simulink model "array_sum"  (R2013b)
settings: Solver=ode45  StartTime=0.0  StopTime=10.0  RelTol=1e-3
settings Model: Creator=Chris  LastModifiedBy=Chris

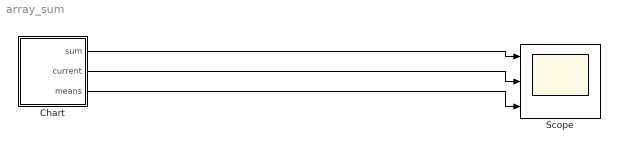
== system array_sum ==
  Chart : Stateflow chart  TreatAsAtomicUnit=on
  Scope : Scope  NumInputPorts=3
      settings: YMin=1~0~-5  YMax=3~7.5~5
  wires:
  Chart/1(sum) -> Scope/1
  Chart/2(current) -> Scope/2
  Chart/3(means) -> Scope/3

== stateflow chart array_sum/Chart ==
  state init
    array[0] = 1;
    array[1] = 2;
    array[2] = 3;
    array[3] = 4;
    array[4] = 5;
    array[5] = 6;
    array[6] = 7;
    array[7] = 8;
    array[8] = 9;
    array[9] = 10;
    array[10] = 11;
    array[11] = 12;
    array[12] = 13;
    length = 13;
    sumCap = 5;
    sum = 0;
  state Rolling_mean
    state Sum_and_Mean
      (junction 54) -> (junction 6) : {i = 0;}
      (junction 6) -> (junction 4) [order 1] : [i < sumCap]
      (junction 4) -> (junction 5) : {sum = sum + array[i + 2*current];}
      (junction 5) -> (junction 6) : {i = i + 1;}
      (junction 6) -> (junction 3) [order 2]
      (junction 3) -> (junction 31) : {means[current] = sum / sumCap;}
    (junction 39) -> (junction 54) [order 1] : [current < (length - (sumCap + 1))]
    (junction 40) -> (junction 39) : {current = 0;}
    (junction 31) -> (junction 39) : {current = current + 1;}
    (junction 39) -> (junction 7) [order 2]
  state Done
  (default) -> init
  init -> (junction 40)
  (junction 7) -> Done
  data: array local double size=100; i local double; sum output double; length local double; current output double; sumCap local double; means output double size=100
